simulink model "robot_diferencial"  (R2024b)
settings: Solver=VariableStepAuto  StartTime=0.0  StopTime=2  RelTol=1e-3
libraries: robotmobilelib x1
settings Model: Creator=usuario  LastModifiedBy=usuario

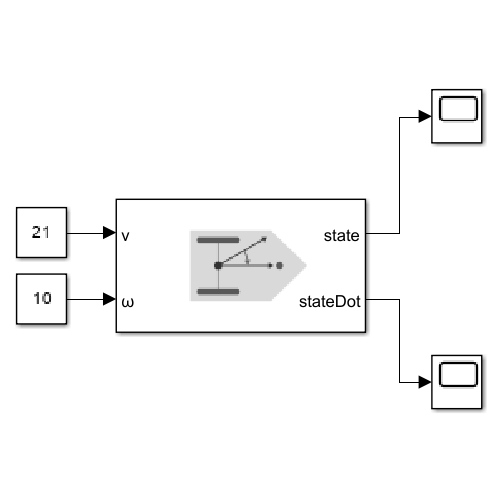
[thumbnail: Simulink's stored preview of the top-level diagram]
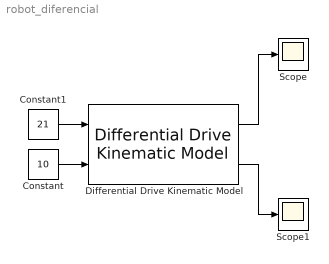
== system robot_diferencial ==
  Constant : Constant  Value=10
  Constant1 : Constant  Value=21
  Differential Drive Kinematic Model : robotmobilelib/Differential Drive Kinematic Model  VehicleInputs=Vehicle Speed & Heading Angular Velocity  WheelRadius=0.05  WheelSpeedRange=[-inf inf]  TrackWidth=0.2  InitialState=[0; 0; 0]  SimulateUsing=Interpreted execution
  Scope : Scope
  Scope1 : Scope
  wires:
  Constant1/1 -> Differential Drive Kinematic Model/1
  Differential Drive Kinematic Model/1 -> Scope/1
  Differential Drive Kinematic Model/2 -> Scope1/1
  Constant/1 -> Differential Drive Kinematic Model/2
